simulink model "ME419_EX1_3"  (R2023b)
settings: Solver=VariableStepAuto  StartTime=0.0  StopTime=10.0  RelTol=1e-6
settings Model: Creator=andyjwaideh  LastModifiedBy=aliawolken

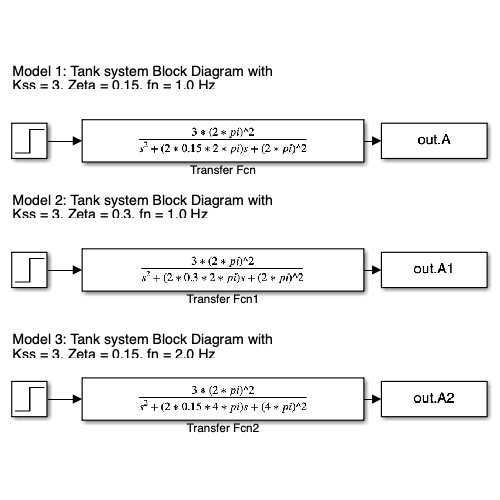
[thumbnail: Simulink's stored preview of the top-level diagram]
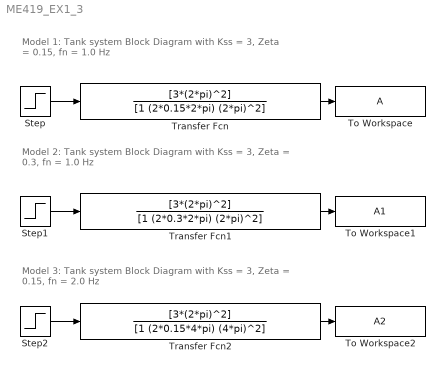
== system ME419_EX1_3 ==
  note: Model 1: Tank system Block Diagram with Kss = 3, Zeta = 0.15, fn = 1.0 Hz
  note: Model 2: Tank system Block Diagram with Kss = 3, Zeta = 0.3, fn = 1.0 Hz
  note: Model 3: Tank system Block Diagram with Kss = 3, Zeta = 0.15, fn = 2.0 Hz
  Step : Step  SampleTime=0
  Step1 : Step  SampleTime=0
  Step2 : Step  SampleTime=0
  To Workspace : ToWorkspace  VariableName=A  SampleTime=-1
  To Workspace1 : ToWorkspace  VariableName=A1  SampleTime=-1
  To Workspace2 : ToWorkspace  VariableName=A2  SampleTime=-1
  Transfer Fcn : TransferFcn  Numerator=[3*(2*pi)^2]  Denominator=[1 (2*0.15*2*pi) (2*pi)^2]
  Transfer Fcn1 : TransferFcn  Numerator=[3*(2*pi)^2]  Denominator=[1 (2*0.3*2*pi) (2*pi)^2]
  Transfer Fcn2 : TransferFcn  Numerator=[3*(2*pi)^2]  Denominator=[1 (2*0.15*4*pi) (4*pi)^2]
  wires:
  Step/1 -> Transfer Fcn/1
  Transfer Fcn/1 -> To Workspace/1
  Step1/1 -> Transfer Fcn1/1
  Transfer Fcn1/1 -> To Workspace1/1
  Step2/1 -> Transfer Fcn2/1
  Transfer Fcn2/1 -> To Workspace2/1
